simulink model "THREE_PHASE_180"  (R2023a)
settings: Solver=VariableStepAuto  StartTime=0.0  StopTime=0.1  MaxStep=1e-5  MinStep=1e-6  RelTol=1e-3
libraries: fl_lib x31, nesl_utility x31, ee_lib x10
settings Model: Creator=admin  LastModifiedBy=admin
settings RTWCC: GPUComputeCapability=5.0

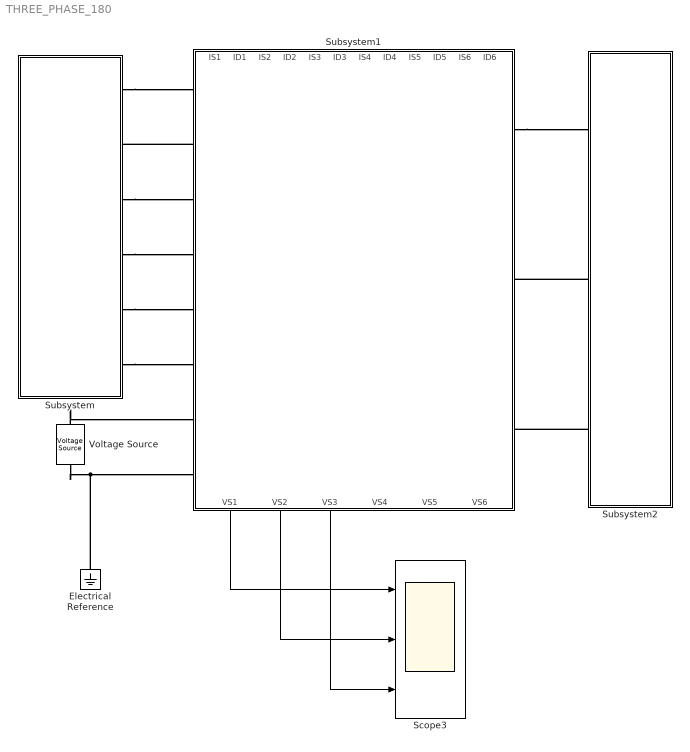
== system THREE_PHASE_180 ==
  Electrical Reference : fl_lib/Electrical/Electrical Elements/Electrical Reference
  Scope3 : Scope  NumInputPorts=3
  Subsystem : Subsystem
  Subsystem1 : Subsystem
      settings: PortSchema="{\"entries\":[{\"content\":{\"sides\":[{\"content\":{\"connectorIds\":[\"LConn1\",\"LConn2\",\"LConn3\"]},\"type\":\"ConnectorPlacement.EquallySpacedRectSide\",\"uuid\":\"5d4c92a2-ca5b-4360-96e8-41c3d64711ed\"},{\"content\":{\"connectorIds\":[\"RConn1\",\"RConn2\",\"RConn3\",\"RConn4\",\"RConn5\",\"RConn6\",\"RConn7\",\"RConn8\"],\"side\":\"RIGHT\"},\"type\":\"ConnectorPlacement.EquallySpacedRectSide\",\"uuid\":\"a457f45b-9620-4720-a303-64053e00b06b\"},{\"content\":{\"connectorIds\":[\"Out13\",\"Out14\",\"Out15\",\"Out16\",\"Out17\",\"Out18\"],\"side\":\"TOP\"},\"type\":\"ConnectorPlacement.EquallySpacedRectSide\",\"uuid\":\"298cbb4c-8ecf-4ea0-bed4-5b126e4f88f2\"},{\"content\":{\"connectorIds\":[\"Out1\",\"Out2\",\"Out3\",\"Out4\",\"Out5\",\"Out6\",\"Out7\",\"Out8\",\"Out9\",\"Out10\",\"Out11\",\"Out12\"],\"side\":\"BOTTOM\"},\"type\":\"ConnectorPlacement.EquallySpacedRectSide\",\"uuid\":\"7f9a027b-cc9b-4311-87e5-9c4d634c220b\"}]},\"type\":\"ConnectorPlacement.EquallySpacedConnector\",\"uuid\":\"e00c9d97-7469-4c00-8f13-230a23b74654\"}],\"packageUris\":[\"http://schema.mathworks.com/mf0/Connector/R2020b\"],\"version\":\"1.0\"}"
  Subsystem2 : Subsystem
  Voltage Source : ee_lib/Sources/Voltage Source  dc_voltage=100 V  ac_voltage=0 V  ac_shift=0 rad  ac_frequency=0 Hz  noise_mode=ee.enum.sources.noise.Disabled  PSD=0 V^2/Hz  sample_time=1e-3 s  repeatability=ee.enum.sources.repeatability.NotRepeatable  user_seed=0  auto_seed=2715962282  i_specify=off  i_priority=None  i=0 A  i_nominal_specify=off  i_nominal_value=1  i_nominal_unit=A  v_specify=off  v_priority=None  v=0 V  v_nominal_specify=off  v_nominal_value=1  v_nominal_unit=V
  wires:
  Subsystem1/18(VS1) -> Scope3/1
  Subsystem1/17(VS2) -> Scope3/2
  Subsystem1/16(VS3) -> Scope3/3
  connections:
  Voltage Source/LConn1 -- Subsystem1/RConn2
  Voltage Source/RConn1 -- Subsystem1/RConn1 -- Electrical Reference/LConn1
  Subsystem/RConn1 -- Subsystem1/RConn8
  Subsystem1/RConn7 -- Subsystem/RConn2
  Subsystem/RConn3 -- Subsystem1/RConn6
  Subsystem/RConn4 -- Subsystem1/RConn5
  Subsystem/RConn5 -- Subsystem1/RConn4
  Subsystem/RConn6 -- Subsystem1/RConn3
  Subsystem2/LConn2 -- Subsystem1/LConn2
  Subsystem1/LConn3 -- Subsystem2/LConn1
  Subsystem2/LConn3 -- Subsystem1/LConn1

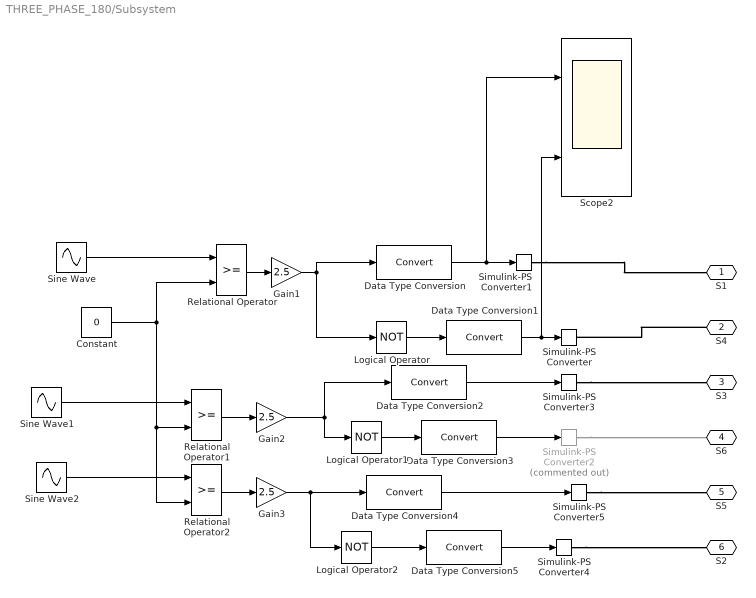
== system THREE_PHASE_180/Subsystem ==
  Constant : Constant  Value=0
  Data Type Conversion{,1..5} (6 alike) : DataTypeConversion  SaturateOnIntegerOverflow=off  RndMeth=Floor
  Gain1 : Gain  Gain=2.5
  Gain2 : Gain  Gain=2.5
  Gain3 : Gain  Gain=2.5
  Logical Operator : Logic  Operator=NOT  AllPortsSameDT=off  OutDataTypeStr=boolean
  Logical Operator1 : Logic  Operator=NOT  AllPortsSameDT=off  OutDataTypeStr=boolean
  Logical Operator2 : Logic  Operator=NOT  AllPortsSameDT=off  OutDataTypeStr=boolean
  Relational Operator : RelationalOperator  OutDataTypeStr=boolean  RndMeth=Simplest  InputSameDT=off
  Relational Operator1 : RelationalOperator  OutDataTypeStr=boolean  RndMeth=Simplest  InputSameDT=off
  Relational Operator2 : RelationalOperator  OutDataTypeStr=boolean  RndMeth=Simplest  InputSameDT=off
  Scope2 : Scope  NumInputPorts=2
  Simulink-PS Converter{,1,3..5} (5 alike) : nesl_utility/Simulink-PS Converter  PhysicalDomain=network_engine_domain  SubClassName=ps_input  LeftPortType=input  RightPortType=output  PseudoPeriodic=off  Frequencies=[]  NoiseDistribution=none  NoiseParameters=[]  Unit=1  AffineConversion=off  FilteringAndDerivatives=provide  SimscapeFilterOrder=1  InputFilterTimeConstant=0.001  UdotUserProvided=0
  Simulink-PS Converter2 : nesl_utility/Simulink-PS Converter  Commented=on  PhysicalDomain=network_engine_domain  SubClassName=ps_input  LeftPortType=input  RightPortType=output  PseudoPeriodic=off  Frequencies=[]  NoiseDistribution=none  NoiseParameters=[]  Unit=1  AffineConversion=off  FilteringAndDerivatives=provide  SimscapeFilterOrder=1  InputFilterTimeConstant=0.001  UdotUserProvided=0
  Sine Wave : Sin  Frequency=2*pi*50  SampleTime=0
  Sine Wave1 : Sin  Frequency=2*pi*50  Phase=2*pi/3  SampleTime=0
  Sine Wave2 : Sin  Frequency=2*pi*50  Phase=-2*pi/3  SampleTime=0
  S1 : PMIOPort  Side=Right
  S4 : PMIOPort  Port=2  Side=Right
  S3 : PMIOPort  Port=3  Side=Right
  S6 : PMIOPort  Port=4  Side=Right
  S5 : PMIOPort  Port=5  Side=Right
  S2 : PMIOPort  Port=6  Side=Right
  wires:
  Constant/1 -> Relational Operator/2, Relational Operator2/2, Relational Operator1/2
  Data Type Conversion/1 -> Scope2/1, Simulink-PS Converter1/1
  Data Type Conversion5/1 -> Simulink-PS Converter4/1
  Data Type Conversion2/1 -> Simulink-PS Converter3/1
  Data Type Conversion1/1 -> Scope2/2, Simulink-PS Converter/1
  Sine Wave2/1 -> Relational Operator2/1
  Gain3/1 -> Logical Operator2/1, Data Type Conversion4/1
  Relational Operator/1 -> Gain1/1
  Sine Wave1/1 -> Relational Operator1/1
  Sine Wave/1 -> Relational Operator/1
  Relational Operator1/1 -> Gain2/1
  Relational Operator2/1 -> Gain3/1
  Logical Operator1/1 -> Data Type Conversion3/1
  Gain2/1 -> Logical Operator1/1, Data Type Conversion2/1
  Logical Operator2/1 -> Data Type Conversion5/1
  Data Type Conversion3/1 -> Simulink-PS Converter2/1
  Gain1/1 -> Data Type Conversion/1, Logical Operator/1
  Logical Operator/1 -> Data Type Conversion1/1
  Data Type Conversion4/1 -> Simulink-PS Converter5/1
  connections:
  S4/RConn1 -- Simulink-PS Converter/RConn1
  Simulink-PS Converter1/RConn1 -- S1/RConn1
  Simulink-PS Converter2/RConn1 -- S6/RConn1
  Simulink-PS Converter4/RConn1 -- S2/RConn1
  Simulink-PS Converter3/RConn1 -- S3/RConn1
  Simulink-PS Converter5/RConn1 -- S5/RConn1

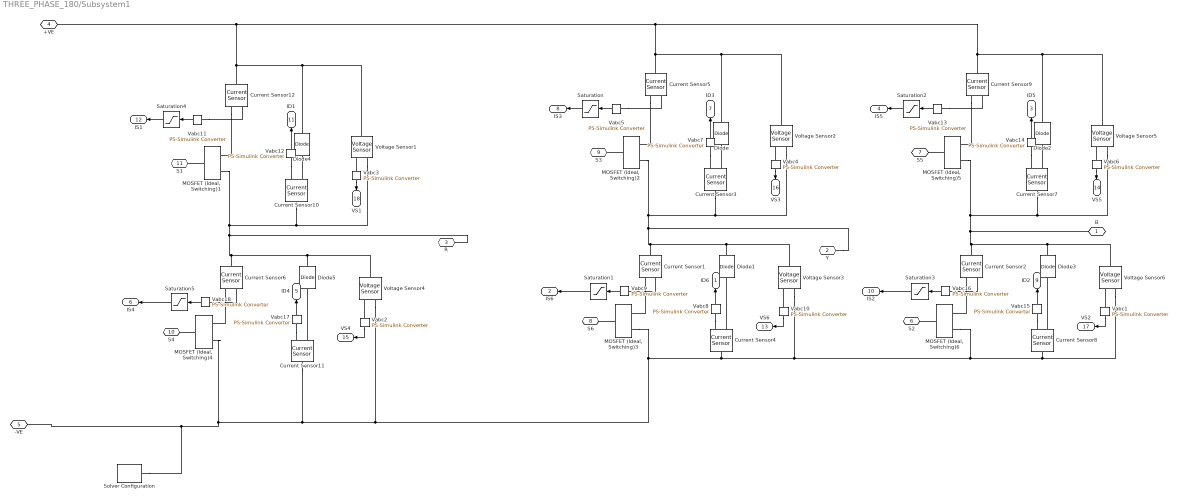
== system THREE_PHASE_180/Subsystem1 ==
  Current Sensor{1..12} (12 alike) : fl_lib/Electrical/Electrical Sensors/Current Sensor
  Diode{,1..5} (6 alike) : fl_lib/Electrical/Electrical Elements/Diode  Vf=0.6 V  Ron=0.3 Ohm  Goff=1e-8 1/Ohm  i_specify=off  i_priority=None  i=0 A  i_nominal_specify=off  i_nominal_value=1  i_nominal_unit=A  v_specify=off  v_priority=None  v=0 V  v_nominal_specify=off  v_nominal_value=1  v_nominal_unit=V
  MOSFET (Ideal, Switching){1..6} (6 alike) : ee_lib/Semiconductors & Converters/MOSFET (Ideal, Switching)  port_option=ee.enum.controlport.ps  Rds=0.01 Ohm  Goff=1e-6 1/Ohm  Vth=2 V  diode_param=ee.enum.converters.protectiondiode.none  diode_Vf=0.8 V  diode_Ron=0.001 Ohm  diode_Goff=1e-5 1/Ohm  diode_C=50e-9 F  diode_iRM=-235 A  diode_iF=300 A  diode_idot=-50 A/us  diode_trr_param=ee.enum.converters.diodeReverseParam.trr_factor  diode_trr_factor=3  diode_trr=15 us  diode_Qrr=1500 s*uA  ids_specify=off  ids_priority=None  ids=0 A  ids_nominal_specify=off  ids_nominal_value=1  ids_nominal_unit=A  vds_specify=off  vds_priority=None  vds=0 V  vds_nominal_specify=off  vds_nominal_value=1  vds_nominal_unit=V  vgs_specify=off  vgs_priority=None  vgs=0 V  vgs_nominal_specify=off  vgs_nominal_value=1  vgs_nominal_unit=V  thermal_loss_option=ee.enum.converters.thermalLossOption.constantvalues  Von_data=[0, 1.8, 3.2, 6, 10, 16; 0, 2, 5.5, 9.5, 15, 25] V  Tj=[298.15, 448.15] K  Iout_data=[0, 20, 40, 60, 80, 100] A  Eon_data=[0, 55.04, 124.57, 235.53, 362.12; 0, 71.25, 161.25, 304.88, 468.75] * 1e-6 J  Eoff_data=[0, 18, 30, 56.1, 76.5; 0, 22.5, 37.5, 70.13, 95.63] * 1e-6 J  Eon_data_3D=[zeros(2, 5, 3)] J  Eoff_data_3D=[zeros(2, 5, 3)] J  Tj_loss=[298.15, 448.15] K  Iout_data_loss=[0, 10, 20, 30, 40] A  tabulateWithVds=false  Vds_loss=[0, 150, 300] V  Eon_scalar=22.86e-3 J  Eoff_scalar=17.14e-3 J  Voff=300 V  Iout_scalar=600 A  useCurrentFromPreviousCycle=false  useVoltageFromPreviousCycle=false  diodeModelType=ee.enum.converters.diodeModelType.pwl  diodeTableType=ee.enum.diode.tableType.IfMat  diode_ReverseIVType=ee.enum.diode.diodeReverseIV.constant  diode_IfMat=[.07, .12, .19, 1.75, 4.24, 7.32, 11.2; .16, .3, .72, 2.14, 4.02, 6.35, 9.12] A  diode_VfMat=[.9, 1.15, 1.25, 1.5, 1.75, 2.17, 2.6, 2.85; .58, .68, .75, 1.1, 1.38, 1.77, 2.27, 2.7] V  diode_TjVec=[25, 125] degC  diode_VfVec=[.5, .7, .9, 1.3, 1.7, 2.1, 2.5] V  diode_IfVec=[.1, .2, .5, 1, 2, 4, 7, 10] A  diode_IrMat=[1e-06, 2e-06, 5e-06, 1e-05, 2.5e-05, 5e-05, .0001; 2e-06, 5e-06, 1e-05, 4e-05, 8e-05, .0002, .0005] A  diode_VrMat=[10, 100, 200, 250, 300, 325, 350; 10, 70, 160, 220, 270, 300, 320] V  diode_VrVec=[10, 20, 40, 50, 70, 80, 100] V  diode_IrVec=[1e-06, 2e-06, 5e-06, 1e-05, 2e-05, 5e-05, .0001] A  diode_Vr=-600 V  diode_Ls=150 nH  diode_Erec=0.03 J  diode_rec_loss_model=ee.enum.diode.reverseRecoveryModel.fixed  diode_ErecVal=0 J  diode_scaleWithIandV=true  diode_ErecMat=zeros(2, 3) J  diode_TjrecVec=[298.15, 398.15] K  diode_IfrecVec=[.1, 1, 10] A  diode_IrecVal=10 A  diode_VrecVal=10 V  diode_tFilter=1 / 1000 / 100 s  thermal_network_parameterization=ee.enum.thermalNetworkTopology.external  Rth=[.03, .2] K/W  Rth_Cauer=[.03, .1, .2] K/W  Rth_Foster=[.03, .2] K/W  thermal_mass_parameterization=ee.enum.thermalNetwork.timeconstant  thermal_mass=[3, 25] J/K  thermal_mass_Cauer=[3, 10, 25] J/K  thermal_mass_Foster=[33, 50] J/K  thermal_time_constant=[.1, 5] s  thermal_time_constant_Cauer=[.1, 1, 5] s  thermal_time_constant_Foster=[1, 10] s  thermal_mass_initial_temperatures=[25, 25] degC  thermal_mass_initial_temperatures_Cauer=[25, 25, 25] degC  junction_thermal_mass=0.1 J/K  Tvec_initial_Foster=[25, 25, 25, 25] degC  no_thermal_network=0  junction_temperature_specify=off  junction_temperature_priority=None  junction_temperature=25 degC  junction_temperature_nominal_specify=off  junction_temperature_nominal_value=1  junction_temperature_nominal_unit=degC  Qj_specify=off  Qj_priority=None  Qj=0 W  Qj_nominal_specify=off  Qj_nominal_value=1  Qj_nominal_unit=W  accumulatedSwitchingLosses_specify=off  accumulatedSwitchingLosses_priority=None  accumulatedSwitchingLosses=0 J
  Saturation{,1..5} (6 alike) : Saturate  UpperLimit=1  LowerLimit=-1
  Solver Configuration : nesl_utility/Solver Configuration  PhysicalDomain=network_engine_domain  SubClassName=solver  LeftPortType=input  RightPortType=generic  Tones=[]  Harmonics=[]  SimulateNoise=off  Profile=off  UseLocalSampling=off  EnableSwitchedLinearOptims=on  FrequencyDomain=off  UseCCode=off  RelTol=0.001  AbsTol=0.001  MinStep=1e-09  ToWorkspace=off  RevertToSquareIcSolve=off  NumHomotopyIterations=100  PhasorMode=off  PhasorModeNumHarmonics=1  ConsistencySolver=NEWTON_FTOL  IndexReductionMethod=DerivativeReplacement  DoDC=off  ResidualTolerance=1e-09  ConsistencyTolSource=GLOBAL  ConsistencyAbsTol=0.001  ConsistencyRelTol=0.001  ConsistencyTolFactor=0.001  UseLocalSolver=off  LocalSolverChoice=NE_BACKWARD_EULER_ADVANCER  ResolveIndetEquations=on  FunctionEvalNumThread=1  LocalSolverSampleTime=0.001  DoFixedCost=off  MaxNonlinIter=3  MaxModeIter=2  ComputeImpulses=off  ImpulseIterations=2  LinearAlgebra=auto  LinearAlgebraNumThread=0  EquationFormulation=NE_TIME_EF  DelaysMemoryBudget=1024  AutomaticFiltering=on  FilteringTimeConstant=0.001  PartitionStorageMethod=AS_NEEDED  PartitionMemoryBudget=1024  PartitionMethod=ROBUST  MultibodyUseLocalSolver=off  MultibodyLocalSolverChoice=ODE1  MultibodyLocalSolverSampleTime=0.001
  Vabc{1..18} (18 alike) : nesl_utility/PS-Simulink Converter  PhysicalDomain=network_engine_domain  SubClassName=ps_output  LeftPortType=input  RightPortType=output  PseudoPeriodic=off  Frequencies=[]  VectorFormat=inherit  Unit=inherit  AffineConversion=off
  Voltage Sensor{1..6} (6 alike) : fl_lib/Electrical/Electrical Sensors/Voltage Sensor
  B : PMIOPort  Side=Left
  Y : PMIOPort  Port=2  Side=Left
  R : PMIOPort  Port=3  Side=Left
  +VE : PMIOPort  Port=4  Side=Right
  -VE : PMIOPort  Port=5  Side=Right
  S2 : PMIOPort  Port=6  Side=Right
  S5 : PMIOPort  Port=7  Side=Right
  S6 : PMIOPort  Port=8  Side=Right
  S3 : PMIOPort  Port=9  Side=Right
  S4 : PMIOPort  Port=10  Side=Right
  S1 : PMIOPort  Port=11  Side=Right
  ID6 : Outport
  IS6 : Outport  Port=2
  ID5 : Outport  Port=3
  IS5 : Outport  Port=4
  ID4 : Outport  Port=5
  IS4 : Outport  Port=6
  ID3 : Outport  Port=7
  IS3 : Outport  Port=8
  ID2 : Outport  Port=9
  IS2 : Outport  Port=10
  ID1 : Outport  Port=11
  IS1 : Outport  Port=12
  VS6 : Outport  Port=13
  VS5 : Outport  Port=14
  VS4 : Outport  Port=15
  VS3 : Outport  Port=16
  VS2 : Outport  Port=17
  VS1 : Outport  Port=18
  wires:
  Vabc4/1 -> VS3/1
  Vabc5/1 -> Saturation/1
  Vabc7/1 -> ID3/1
  Vabc8/1 -> ID6/1
  Saturation/1 -> IS3/1
  Vabc9/1 -> Saturation1/1
  Saturation1/1 -> IS6/1
  Vabc10/1 -> VS6/1
  Vabc1/1 -> VS2/1
  Saturation3/1 -> IS2/1
  Saturation2/1 -> IS5/1
  Vabc16/1 -> Saturation3/1
  Vabc14/1 -> ID5/1
  Vabc15/1 -> ID2/1
  Vabc6/1 -> VS5/1
  Vabc13/1 -> Saturation2/1
  Vabc2/1 -> VS4/1
  Saturation5/1 -> IS4/1
  Saturation4/1 -> IS1/1
  Vabc18/1 -> Saturation5/1
  Vabc12/1 -> ID1/1
  Vabc17/1 -> ID4/1
  Vabc3/1 -> VS1/1
  Vabc11/1 -> Saturation4/1
  connections:
  Current Sensor8/LConn1 -- Voltage Sensor4/RConn2 -- Current Sensor11/LConn1 -- "MOSFET (Ideal, Switching)4"/RConn2 -- -VE/RConn1 -- Solver Configuration/RConn1 -- "MOSFET (Ideal, Switching)3"/RConn2 -- Current Sensor4/LConn1 -- Voltage Sensor3/RConn2 -- "MOSFET (Ideal, Switching)6"/RConn2 -- Voltage Sensor6/RConn2
  Current Sensor3/LConn1 -- Voltage Sensor2/RConn2 -- Y/RConn1 -- Voltage Sensor3/LConn1 -- Diode1/RConn1 -- Current Sensor1/LConn1 -- "MOSFET (Ideal, Switching)2"/RConn2
  Vabc4/LConn1 -- Voltage Sensor2/RConn1
  "MOSFET (Ideal, Switching)2"/LConn1 -- S3/RConn1
  "MOSFET (Ideal, Switching)3"/LConn1 -- S6/RConn1
  Current Sensor3/RConn2 -- Diode/LConn1
  Current Sensor4/RConn2 -- Diode1/LConn1
  Vabc7/LConn1 -- Current Sensor3/RConn1
  Vabc8/LConn1 -- Current Sensor4/RConn1
  Current Sensor5/RConn2 -- "MOSFET (Ideal, Switching)2"/RConn1
  Vabc5/LConn1 -- Current Sensor5/RConn1
  Vabc9/LConn1 -- Current Sensor1/RConn1
  Current Sensor1/RConn2 -- "MOSFET (Ideal, Switching)3"/RConn1
  Vabc10/LConn1 -- Voltage Sensor3/RConn1
  Current Sensor2/LConn1 -- Current Sensor7/LConn1 -- Voltage Sensor5/RConn2 -- "MOSFET (Ideal, Switching)5"/RConn2 -- B/RConn1 -- Voltage Sensor6/LConn1 -- Diode3/RConn1
  Current Sensor12/LConn1 -- +VE/RConn1 -- Current Sensor9/LConn1 -- Voltage Sensor5/LConn1 -- Diode2/RConn1 -- Current Sensor5/LConn1 -- Voltage Sensor2/LConn1 -- Diode/RConn1 -- Voltage Sensor1/LConn1 -- Diode4/RConn1
  Vabc16/LConn1 -- Current Sensor2/RConn1
  "MOSFET (Ideal, Switching)6"/LConn1 -- S2/RConn1
  Vabc1/LConn1 -- Voltage Sensor6/RConn1
  Current Sensor2/RConn2 -- "MOSFET (Ideal, Switching)6"/RConn1
  Vabc14/LConn1 -- Current Sensor7/RConn1
  Current Sensor7/RConn2 -- Diode2/LConn1
  Vabc13/LConn1 -- Current Sensor9/RConn1
  Current Sensor9/RConn2 -- "MOSFET (Ideal, Switching)5"/RConn1
  Current Sensor8/RConn2 -- Diode3/LConn1
  Vabc6/LConn1 -- Voltage Sensor5/RConn1
  Vabc15/LConn1 -- Current Sensor8/RConn1
  "MOSFET (Ideal, Switching)5"/LConn1 -- S5/RConn1
  Current Sensor6/LConn1 -- "MOSFET (Ideal, Switching)1"/RConn2 -- Current Sensor10/LConn1 -- Voltage Sensor1/RConn2 -- R/RConn1 -- Voltage Sensor4/LConn1 -- Diode5/RConn1
  Vabc18/LConn1 -- Current Sensor6/RConn1
  "MOSFET (Ideal, Switching)4"/LConn1 -- S4/RConn1
  Current Sensor6/RConn2 -- "MOSFET (Ideal, Switching)4"/RConn1
  Vabc12/LConn1 -- Current Sensor10/RConn1
  Current Sensor10/RConn2 -- Diode4/LConn1
  Current Sensor12/RConn2 -- "MOSFET (Ideal, Switching)1"/RConn1
  Vabc11/LConn1 -- Current Sensor12/RConn1
  "MOSFET (Ideal, Switching)1"/LConn1 -- S1/RConn1
  Vabc3/LConn1 -- Voltage Sensor1/RConn1
  Vabc2/LConn1 -- Voltage Sensor4/RConn1
  Vabc17/LConn1 -- Current Sensor11/RConn1
  Current Sensor11/RConn2 -- Diode5/LConn1

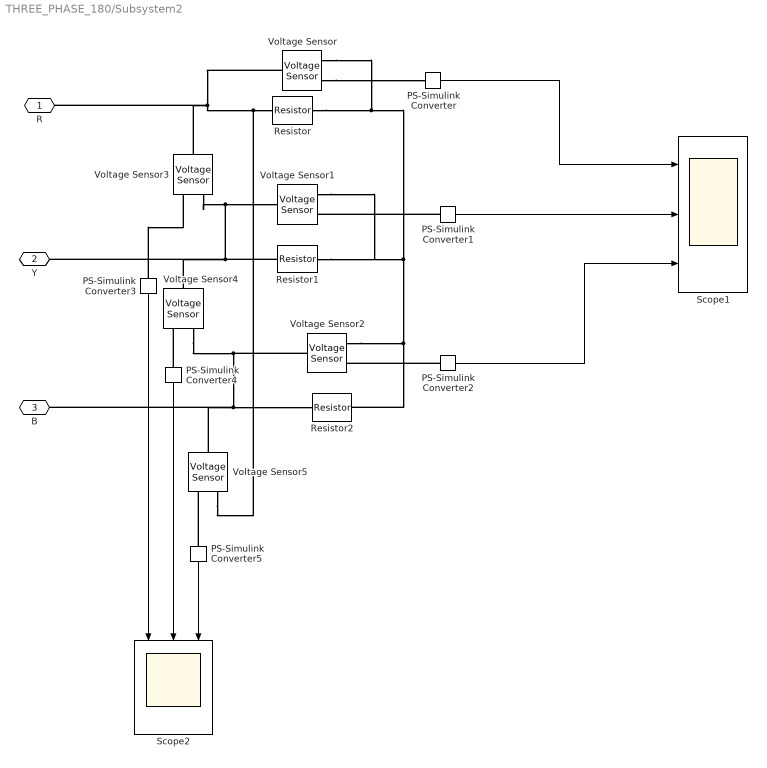
== system THREE_PHASE_180/Subsystem2 ==
  PS-Simulink Converter{,1..5} (6 alike) : nesl_utility/PS-Simulink Converter  PhysicalDomain=network_engine_domain  SubClassName=ps_output  LeftPortType=input  RightPortType=output  PseudoPeriodic=off  Frequencies=[]  VectorFormat=inherit  Unit=inherit  AffineConversion=off
  Resistor : ee_lib/Passive/Resistor  R=100 Ohm  enable_R_tol=ee.enum.toleranceApplication.none  R_tol=5  tol_distribution=ee.enum.toleranceDistribution.uniform  nSigma=4  enable_operating_limits=ee.enum.enable.no  operating_limit_action=ee.enum.passive.reportOpLim.warn  power_rating=1 W  max_working_voltage=100 V  enable_faults=ee.enum.enable.no  fault_action=simscape.enum.assert.action.none  R_faulted=inf Ohm  fault_trigger=ee.enum.faults.faultTrigger.temporal  t_fault=1 s  max_permissible_current=1 A  t_fail_on_current=1 s  noise_mode=ee.enum.sources.noise.Disabled  Tdevice=25 degC  sample_time=1e-3 s  repeatability=ee.enum.ic.repeatability.notRepeatable  user_seed=0  auto_seed=3890346746  faulted_specify=off  faulted_priority=None  faulted=0  power_derating_T1=70 degC  power_derating_T2=155 degC  operating_temperature_range_vec=[-50, 150] degC  alpha=3.93e-3 1/K  Tmeas=25 degC  thermal_mass=100 J/K  temperature_specify=off  temperature_priority=High  temperature=298.15 K  temperature_nominal_specify=off  temperature_nominal_value=1  temperature_nominal_unit=K
  Resistor1 : ee_lib/Passive/Resistor  R=100 Ohm  enable_R_tol=ee.enum.toleranceApplication.none  R_tol=5  tol_distribution=ee.enum.toleranceDistribution.uniform  nSigma=4  enable_operating_limits=ee.enum.enable.no  operating_limit_action=ee.enum.passive.reportOpLim.warn  power_rating=1 W  max_working_voltage=100 V  enable_faults=ee.enum.enable.no  fault_action=simscape.enum.assert.action.none  R_faulted=inf Ohm  fault_trigger=ee.enum.faults.faultTrigger.temporal  t_fault=1 s  max_permissible_current=1 A  t_fail_on_current=1 s  noise_mode=ee.enum.sources.noise.Disabled  Tdevice=25 degC  sample_time=1e-3 s  repeatability=ee.enum.ic.repeatability.notRepeatable  user_seed=0  auto_seed=545404223  faulted_specify=off  faulted_priority=None  faulted=0  power_derating_T1=70 degC  power_derating_T2=155 degC  operating_temperature_range_vec=[-50, 150] degC  alpha=3.93e-3 1/K  Tmeas=25 degC  thermal_mass=100 J/K  temperature_specify=off  temperature_priority=High  temperature=298.15 K  temperature_nominal_specify=off  temperature_nominal_value=1  temperature_nominal_unit=K
  Resistor2 : ee_lib/Passive/Resistor  R=100 Ohm  enable_R_tol=ee.enum.toleranceApplication.none  R_tol=5  tol_distribution=ee.enum.toleranceDistribution.uniform  nSigma=4  enable_operating_limits=ee.enum.enable.no  operating_limit_action=ee.enum.passive.reportOpLim.warn  power_rating=1 W  max_working_voltage=100 V  enable_faults=ee.enum.enable.no  fault_action=simscape.enum.assert.action.none  R_faulted=inf Ohm  fault_trigger=ee.enum.faults.faultTrigger.temporal  t_fault=1 s  max_permissible_current=1 A  t_fail_on_current=1 s  noise_mode=ee.enum.sources.noise.Disabled  Tdevice=25 degC  sample_time=1e-3 s  repeatability=ee.enum.ic.repeatability.notRepeatable  user_seed=0  auto_seed=3922919431  faulted_specify=off  faulted_priority=None  faulted=0  power_derating_T1=70 degC  power_derating_T2=155 degC  operating_temperature_range_vec=[-50, 150] degC  alpha=3.93e-3 1/K  Tmeas=25 degC  thermal_mass=100 J/K  temperature_specify=off  temperature_priority=High  temperature=298.15 K  temperature_nominal_specify=off  temperature_nominal_value=1  temperature_nominal_unit=K
  Scope1 : Scope  NumInputPorts=3
  Scope2 : Scope  NumInputPorts=3
  Voltage Sensor{,1..5} (6 alike) : fl_lib/Electrical/Electrical Sensors/Voltage Sensor
  R : PMIOPort  Side=Left
  Y : PMIOPort  Port=2  Side=Left
  B : PMIOPort  Port=3  Side=Left
  wires:
  PS-Simulink Converter5/1 -> Scope2/3
  PS-Simulink Converter2/1 -> Scope1/3
  PS-Simulink Converter3/1 -> Scope2/1
  PS-Simulink Converter/1 -> Scope1/1
  PS-Simulink Converter4/1 -> Scope2/2
  PS-Simulink Converter1/1 -> Scope1/2
  connections:
  PS-Simulink Converter3/LConn1 -- Voltage Sensor3/RConn1
  Resistor1/LConn1 -- Voltage Sensor4/LConn1 -- Y/RConn1 -- Voltage Sensor1/LConn1 -- Voltage Sensor3/RConn2
  PS-Simulink Converter2/LConn1 -- Voltage Sensor2/RConn1
  PS-Simulink Converter5/LConn1 -- Voltage Sensor5/RConn1
  Voltage Sensor2/LConn1 -- Voltage Sensor4/RConn2 -- B/RConn1 -- Voltage Sensor5/LConn1 -- Resistor2/LConn1
  Voltage Sensor/LConn1 -- R/RConn1 -- Voltage Sensor3/LConn1 -- Resistor/LConn1 -- Voltage Sensor5/RConn2
  PS-Simulink Converter4/LConn1 -- Voltage Sensor4/RConn1
  Resistor/RConn1 -- Voltage Sensor/RConn2 -- Voltage Sensor1/RConn2 -- Resistor1/RConn1 -- Resistor2/RConn1 -- Voltage Sensor2/RConn2
  Voltage Sensor/RConn1 -- PS-Simulink Converter/LConn1
  PS-Simulink Converter1/LConn1 -- Voltage Sensor1/RConn1
